simulink model "Subtractor"  (R2018a)
settings: Solver=VariableStepAuto  StartTime=0.0  StopTime=10.0  RelTol=1e-3
settings Model: Creator=midog  LastModifiedBy=midog

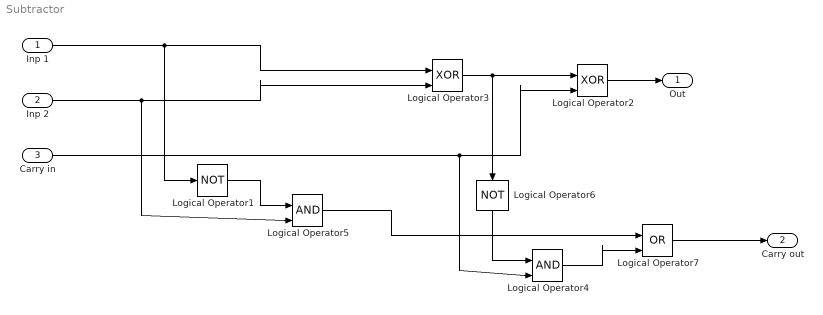
== system Subtractor ==
  Inp 1 : Inport
  Inp 2 : Inport  Port=2
  Carry in : Inport  Port=3
  Logical Operator1 : Logic  Operator=NOT  IconShape=distinctive  AllPortsSameDT=off  OutDataTypeStr=boolean
  Logical Operator2 : Logic  Operator=XOR  IconShape=distinctive  AllPortsSameDT=off  OutDataTypeStr=boolean
  Logical Operator3 : Logic  Operator=XOR  IconShape=distinctive  AllPortsSameDT=off  OutDataTypeStr=boolean
  Logical Operator4 : Logic  IconShape=distinctive  AllPortsSameDT=off  OutDataTypeStr=boolean
  Logical Operator5 : Logic  IconShape=distinctive  AllPortsSameDT=off  OutDataTypeStr=boolean
  Logical Operator6 : Logic  Operator=NOT  IconShape=distinctive  AllPortsSameDT=off  OutDataTypeStr=boolean
  Logical Operator7 : Logic  Operator=OR  IconShape=distinctive  AllPortsSameDT=off  OutDataTypeStr=boolean
  Out : Outport
  Carry out : Outport  Port=2
  wires:
  Logical Operator7/1 -> Carry out/1
  Logical Operator5/1 -> Logical Operator7/1
  Carry in/1 -> Logical Operator4/2, Logical Operator2/2
  Logical Operator1/1 -> Logical Operator5/1
  Logical Operator6/1 -> Logical Operator4/1
  Inp 2/1 -> Logical Operator5/2, Logical Operator3/2
  Inp 1/1 -> Logical Operator1/1, Logical Operator3/1
  Logical Operator4/1 -> Logical Operator7/2
  Logical Operator3/1 -> Logical Operator6/1, Logical Operator2/1
  Logical Operator2/1 -> Out/1
